simulink model "tp2segway"  (R2020b)
settings: Solver=FixedStepAuto  StartTime=0.0  StopTime=10.0  RelTol=1e-3  EnableMultiTasking=on
values from neighbouring files (symbols this model uses):
  Ts = 0.004    [model.m]
libraries: legoev3lib x5
settings Model: ExtModeTrigDuration=2  Creator=groupe3-2  LastModifiedBy=groupe3-2
settings SolverCC: PositivePriorityOrder=on
settings OptimizationCC: EnhancedBackFolding=on  PassReuseOutputArgsAs=Individual arguments  ZeroExternalMemoryAtStartup=off  ZeroInternalMemoryAtStartup=off  MaxStackSize=64  OptimizeBlockOrder=speed  DifferentSizesBufferReuse=on  OptimizationCustomize=off  EfficientTunableParamExpr=on
settings DebuggingCC: ParameterTunabilityLossMsg=error
settings HardwareCC: ProdBitPerPointer=32  ProdBitPerSizeT=32  ProdBitPerPtrDiffT=32  ProdLargestAtomicInteger=Long  ProdWordSize=32  ProdHWDeviceType=ARM Compatible->ARM 9
settings SFSimCC: MATLABDynamicMemAlloc=off
settings RTWCC: Description=Embedded Coder  SystemTargetFile=ert.tlc  HardwareBoard=LEGO MINDSTORMS EV3  TLCOptions="-aInlineSetEventsForThisBaseRateFcn=TLC_FALSE -aSuppressMultiTaskScheduler=TLC_FALSE  -aRateBasedStepFcn=0"  TemplateMakefile=ert_default_tmf  Toolchain=Sourcery G++ Lite v2009q3
settings CodeAppCC: ForceParamTrailComments=on  IgnoreCustomStorageClasses=off  OperatorAnnotations=on  SimulinkDataObjDesc=on  SFDataObjDesc=on  InsertBlockDesc=on
settings ERTTargetCC: SupportContinuousTime=on  SupportVariableSizeSignals=on  ExtModeTransport=2  ExtModeMexFile=ext_xcp  ExtModeIntrfLevel=Level2 - Open

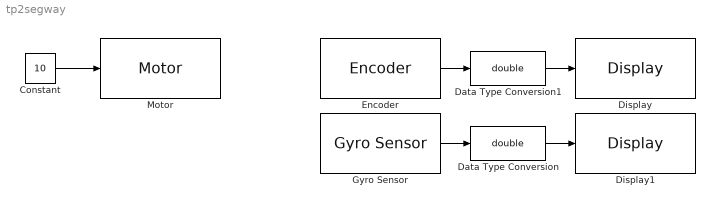
== system tp2segway ==
  Constant : Constant  Value=10  SampleTime=Ts
  Data Type Conversion : DataTypeConversion  OutDataTypeStr=double
  Data Type Conversion1 : DataTypeConversion  OutDataTypeStr=double
  Display : legoev3lib/Display  slcdLine=1  slcdFormat=Decimal
      settings: SourceProductBaseCode=LEGOEV3
  Display1 : legoev3lib/Display  slcdLine=2  slcdFormat=Decimal
      settings: SourceProductBaseCode=LEGOEV3
  Encoder : legoev3lib/Encoder  portNumber=A  opMode=Reset by external signal  sampleTime=Ts
      settings: SourceProductBaseCode=LEGOEV3
  Gyro Sensor : legoev3lib/Gyro Sensor  portNumber=2  sampleTime=Ts
      settings: SourceProductBaseCode=LEGOEV3
  Motor : legoev3lib/Motor  sportNumber=A  sstopAction=Brake
  wires:
  Constant/1 -> Motor/1
  Encoder/1 -> Data Type Conversion1/1
  Data Type Conversion1/1 -> Display/1
  Gyro Sensor/1 -> Data Type Conversion/1
  Data Type Conversion/1 -> Display1/1
